simulink model "HVDCMMCInterconnection"  (R2023b)
settings: Solver=FixedStepDiscrete  StartTime=0.0  StopTime=10  FixedStep=Ts_Power  RelTol=1e-4
PreLoadFcn:
  | HVDCMMCInterconnectionParam
StartFcn:
  | tic
StopFcn:
  | toc
values from neighbouring files (symbols this model uses):
  C_PM = 1.758e-3    (= 0.001758)    [HVDCMMCInterconnectionParam.m]
  Cg = 50e-9    (= 5e-08)    [HVDCMMCInterconnectionParam.m]
  D_R = 0.001    [HVDCMMCInterconnectionParam.m]
  D_Rs = 1e8    (= 100000000)    [HVDCMMCInterconnectionParam.m]
  D_Vf = 0    [HVDCMMCInterconnectionParam.m]
  Fnom = 50    [HVDCMMCInterconnectionParam.m]
  HRM = 2    [HVDCMMCInterconnectionParam.m]
  Ki_Ireg = 6    [HVDCMMCInterconnectionParam.m]
  Ki_Preg = 1.0    (= 1)    [HVDCMMCInterconnectionParam.m]
  Ki_Qreg = 1.0    (= 1)    [HVDCMMCInterconnectionParam.m]
  Ki_VDCreg = 100    [HVDCMMCInterconnectionParam.m]
  Kp_Ireg = 0.6    [HVDCMMCInterconnectionParam.m]
  Kp_Preg = 0.5/3    (= 0.166666666667)    [HVDCMMCInterconnectionParam.m]
  Kp_Qreg = 0.5/3    (= 0.166666666667)    [HVDCMMCInterconnectionParam.m]
  Kp_VDCreg = 4    [HVDCMMCInterconnectionParam.m]
  L_cable = 15e-3    (= 0.015)    [HVDCMMCInterconnectionParam.m]
  Larm = Larm_pu*(Zb_ac/(2*pi*Fnom))    [HVDCMMCInterconnectionParam.m]
  Lff = Larm_pu/2    (= 0.075)    [HVDCMMCInterconnectionParam.m]
  Limits_Ireg = [ 2.0  -2.0]    [HVDCMMCInterconnectionParam.m]
  Limits_Preg = [ 1.2, 0.8 ]    [HVDCMMCInterconnectionParam.m]
  Limits_Qreg = [ 0.25, -0.25 ]    [HVDCMMCInterconnectionParam.m]
  Limits_VDCreg = [ 2.0  -2.0]    [HVDCMMCInterconnectionParam.m]
  Lxfo = 0.12    [HVDCMMCInterconnectionParam.m]
  Nb_PM = 36    [HVDCMMCInterconnectionParam.m]
  Pnom = 1000e6    (= 1000000000)    [HVDCMMCInterconnectionParam.m]
  R_cable = 0.5    [HVDCMMCInterconnectionParam.m]
  R_startup = 400    [HVDCMMCInterconnectionParam.m]
  Rarm = Rarm_pu*Zb_ac    [HVDCMMCInterconnectionParam.m]
  Rff = Rarm_pu/2    (= 0.00075)    [HVDCMMCInterconnectionParam.m]
  Rg = 100    [HVDCMMCInterconnectionParam.m]
  Rxfo = 0.003    [HVDCMMCInterconnectionParam.m]
  Slope_Pref = 0.5    [HVDCMMCInterconnectionParam.m]
  Slope_Qref = 0.5    [HVDCMMCInterconnectionParam.m]
  Slope_Vdc_ref = Vnom_dc/5    (= 128000)    [HVDCMMCInterconnectionParam.m]
  Tbrk1_On = 0.1    [HVDCMMCInterconnectionParam.m]
  Tbrk2_On = 1.0    (= 1)    [HVDCMMCInterconnectionParam.m]
  Tdeblock = 1.5    [HVDCMMCInterconnectionParam.m]
  Tfault = 9999    [HVDCMMCInterconnectionParam.m]
  Ton_Converter2 = 4    [HVDCMMCInterconnectionParam.m]
  Ton_PQreg = 4    [HVDCMMCInterconnectionParam.m]
  Ton_VDCreg = 1.5    [HVDCMMCInterconnectionParam.m]
  Ts = Ts_Control    (= 4e-05)    [HVDCMMCInterconnectionParam.m]    (also in power_circ2ss_sps_calc.m = 1e-06)
  Ts_Control = 40e-6    (= 4e-05)    [HVDCMMCInterconnectionParam.m]
  Ts_Power = 20e-6    (= 2e-05)    [HVDCMMCInterconnectionParam.m]
  Vb_ac = sqrt(2/3)*Vnom_sec    [HVDCMMCInterconnectionParam.m]
  Vb_dc = Vnom_dc    (= 640000)    [HVDCMMCInterconnectionParam.m]
  Vc0_PM = 0    [HVDCMMCInterconnectionParam.m]
  Vnom_dc = 640e3    (= 640000)    [HVDCMMCInterconnectionParam.m]
  Vnom_prim = 400e3    (= 400000)    [HVDCMMCInterconnectionParam.m]
  Vnom_sec = 333e3    (= 333000)    [HVDCMMCInterconnectionParam.m]
  w = 2*pi*Fnom    (= 314.159265359)    [HVDCMMCInterconnectionParam.m]
undefined symbols (not defined in the file or in its folder): ACDC, ACDC3, DiscIntNeverNeededParam, gcbh, Pcc, S, sps_AC, sps_rtmsupport
libraries: simulink x61, spsControlledVoltageSourceLib x56, spsCurrentMeasurementLib x56, spsDiodeLib x40, spsSeriesRLCBranchLib x32, spsVoltageMeasurementLib x20, powerlib_extras x9, spsHalfBridgeMMCmodel x8, spsGroundLib x7, spsSecondOrderFilterLib x6, spsabctodq0Lib x6, spsMeanLib x3
(part 11 of 11)

== system HVDCMMCInterconnection/DSS1/U-I3/MUX1 ==
  In1 : Inport
  In2 : Inport  Port=2
  Demux4 : Demux  Outputs=3
  Demux5 : Demux  Outputs=3
  Mux13 : Mux  Inputs=2
  Mux14 : Mux  Inputs=2
  Mux15 : Mux  Inputs=3
  Mux8 : Mux  Inputs=2
  Sum1 : Sum  Inputs=1  InputSameDT=on  SaturateOnIntegerOverflow=on  OutDataTypeStr=Inherit: Same as first input
  Sum4 : Sum  Inputs=1  InputSameDT=on  SaturateOnIntegerOverflow=on  OutDataTypeStr=Inherit: Same as first input
  Sum5 : Sum  Inputs=1  InputSameDT=on  SaturateOnIntegerOverflow=on  OutDataTypeStr=Inherit: Same as first input
  UBrk1_EMT : Outport
  wires:
  Demux5/3 -> Mux14/2
  In1/1 -> Demux4/1
  Demux4/1 -> Mux8/1
  Demux5/1 -> Mux8/2
  In2/1 -> Demux5/1
  Sum1/1 -> Mux15/1
  Demux5/2 -> Mux13/2
  Mux14/1 -> Sum5/1
  Mux8/1 -> Sum1/1
  Demux4/2 -> Mux13/1
  Mux13/1 -> Sum4/1
  Sum5/1 -> Mux15/3
  Sum4/1 -> Mux15/2
  Demux4/3 -> Mux14/1
  Mux15/1 -> UBrk1_EMT/1

== system HVDCMMCInterconnection/DSS1/U-I3/MUX2 ==
  In1 : Inport
  In2 : Inport  Port=2
  Demux4 : Demux  Outputs=3
  Demux5 : Demux  Outputs=3
  Mux13 : Mux  Inputs=2
  Mux14 : Mux  Inputs=2
  Mux15 : Mux  Inputs=3
  Mux8 : Mux  Inputs=2
  Sum1 : Sum  Inputs=1  InputSameDT=on  SaturateOnIntegerOverflow=on  OutDataTypeStr=Inherit: Same as first input
  Sum4 : Sum  Inputs=1  InputSameDT=on  SaturateOnIntegerOverflow=on  OutDataTypeStr=Inherit: Same as first input
  Sum5 : Sum  Inputs=1  InputSameDT=on  SaturateOnIntegerOverflow=on  OutDataTypeStr=Inherit: Same as first input
  UBrk1_EMT : Outport
  wires:
  Demux5/3 -> Mux14/2
  In1/1 -> Demux4/1
  Demux4/1 -> Mux8/1
  Demux5/1 -> Mux8/2
  In2/1 -> Demux5/1
  Sum1/1 -> Mux15/1
  Demux5/2 -> Mux13/2
  Mux14/1 -> Sum5/1
  Mux8/1 -> Sum1/1
  Demux4/2 -> Mux13/1
  Mux13/1 -> Sum4/1
  Sum5/1 -> Mux15/3
  Sum4/1 -> Mux15/2
  Demux4/3 -> Mux14/1
  Mux15/1 -> UBrk1_EMT/1

== system HVDCMMCInterconnection/DSS2/BRK_CTRL1/MUX2 ==
  In1 : Inport
  In2 : Inport  Port=2
  Demux4 : Demux  Outputs=3
  Demux5 : Demux  Outputs=3
  Mux13 : Mux  Inputs=2
  Mux14 : Mux  Inputs=2
  Mux15 : Mux  Inputs=3
  Mux8 : Mux  Inputs=2
  Sum1 : Sum  Inputs=1  InputSameDT=on  SaturateOnIntegerOverflow=on  OutDataTypeStr=Inherit: Same as first input
  Sum4 : Sum  Inputs=1  InputSameDT=on  SaturateOnIntegerOverflow=on  OutDataTypeStr=Inherit: Same as first input
  Sum5 : Sum  Inputs=1  InputSameDT=on  SaturateOnIntegerOverflow=on  OutDataTypeStr=Inherit: Same as first input
  Out1 : Outport
  wires:
  Demux5/3 -> Mux14/2
  In1/1 -> Demux4/1
  Demux4/1 -> Mux8/1
  Demux5/1 -> Mux8/2
  In2/1 -> Demux5/1
  Sum1/1 -> Mux15/1
  Demux5/2 -> Mux13/2
  Mux14/1 -> Sum5/1
  Mux8/1 -> Sum1/1
  Demux4/2 -> Mux13/1
  Mux13/1 -> Sum4/1
  Sum5/1 -> Mux15/3
  Sum4/1 -> Mux15/2
  Demux4/3 -> Mux14/1
  Mux15/1 -> Out1/1

== system HVDCMMCInterconnection/DSS2/BRK_CTRL3/MUX2 ==
  In1 : Inport
  In2 : Inport  Port=2
  Demux4 : Demux  Outputs=3
  Demux5 : Demux  Outputs=3
  Mux13 : Mux  Inputs=2
  Mux14 : Mux  Inputs=2
  Mux15 : Mux  Inputs=3
  Mux8 : Mux  Inputs=2
  Sum1 : Sum  Inputs=1  InputSameDT=on  SaturateOnIntegerOverflow=on  OutDataTypeStr=Inherit: Same as first input
  Sum4 : Sum  Inputs=1  InputSameDT=on  SaturateOnIntegerOverflow=on  OutDataTypeStr=Inherit: Same as first input
  Sum5 : Sum  Inputs=1  InputSameDT=on  SaturateOnIntegerOverflow=on  OutDataTypeStr=Inherit: Same as first input
  Out1 : Outport
  wires:
  Demux5/3 -> Mux14/2
  In1/1 -> Demux4/1
  Demux4/1 -> Mux8/1
  Demux5/1 -> Mux8/2
  In2/1 -> Demux5/1
  Sum1/1 -> Mux15/1
  Demux5/2 -> Mux13/2
  Mux14/1 -> Sum5/1
  Mux8/1 -> Sum1/1
  Demux4/2 -> Mux13/1
  Mux13/1 -> Sum4/1
  Sum5/1 -> Mux15/3
  Sum4/1 -> Mux15/2
  Demux4/3 -> Mux14/1
  Mux15/1 -> Out1/1

== system HVDCMMCInterconnection/DSS2/U-I1/MUX1 ==
  In1 : Inport
  In2 : Inport  Port=2
  Demux4 : Demux  Outputs=3
  Demux5 : Demux  Outputs=3
  Mux13 : Mux  Inputs=2
  Mux14 : Mux  Inputs=2
  Mux15 : Mux  Inputs=3
  Mux8 : Mux  Inputs=2
  Sum1 : Sum  Inputs=1  InputSameDT=on  SaturateOnIntegerOverflow=on  OutDataTypeStr=Inherit: Same as first input
  Sum4 : Sum  Inputs=1  InputSameDT=on  SaturateOnIntegerOverflow=on  OutDataTypeStr=Inherit: Same as first input
  Sum5 : Sum  Inputs=1  InputSameDT=on  SaturateOnIntegerOverflow=on  OutDataTypeStr=Inherit: Same as first input
  UBrk1_EMT : Outport
  wires:
  Demux5/3 -> Mux14/2
  In1/1 -> Demux4/1
  Demux4/1 -> Mux8/1
  Demux5/1 -> Mux8/2
  In2/1 -> Demux5/1
  Sum1/1 -> Mux15/1
  Demux5/2 -> Mux13/2
  Mux14/1 -> Sum5/1
  Mux8/1 -> Sum1/1
  Demux4/2 -> Mux13/1
  Mux13/1 -> Sum4/1
  Sum5/1 -> Mux15/3
  Sum4/1 -> Mux15/2
  Demux4/3 -> Mux14/1
  Mux15/1 -> UBrk1_EMT/1

== system HVDCMMCInterconnection/DSS2/U-I1/MUX2 ==
  In1 : Inport
  In2 : Inport  Port=2
  Demux4 : Demux  Outputs=3
  Demux5 : Demux  Outputs=3
  Mux13 : Mux  Inputs=2
  Mux14 : Mux  Inputs=2
  Mux15 : Mux  Inputs=3
  Mux8 : Mux  Inputs=2
  Sum1 : Sum  Inputs=1  InputSameDT=on  SaturateOnIntegerOverflow=on  OutDataTypeStr=Inherit: Same as first input
  Sum4 : Sum  Inputs=1  InputSameDT=on  SaturateOnIntegerOverflow=on  OutDataTypeStr=Inherit: Same as first input
  Sum5 : Sum  Inputs=1  InputSameDT=on  SaturateOnIntegerOverflow=on  OutDataTypeStr=Inherit: Same as first input
  UBrk1_EMT : Outport
  wires:
  Demux5/3 -> Mux14/2
  In1/1 -> Demux4/1
  Demux4/1 -> Mux8/1
  Demux5/1 -> Mux8/2
  In2/1 -> Demux5/1
  Sum1/1 -> Mux15/1
  Demux5/2 -> Mux13/2
  Mux14/1 -> Sum5/1
  Mux8/1 -> Sum1/1
  Demux4/2 -> Mux13/1
  Mux13/1 -> Sum4/1
  Sum5/1 -> Mux15/3
  Sum4/1 -> Mux15/2
  Demux4/3 -> Mux14/1
  Mux15/1 -> UBrk1_EMT/1

== system HVDCMMCInterconnection/DSS2/U-I2/BRK_CTRL3 ==
  UBrk1_EMT : Inport
  Brk_ON : Inport  Port=2
  Cast To Double{,1..3} (4 alike) : DataTypeConversion  OutDataTypeStr=double  SaturateOnIntegerOverflow=off  RndMeth=Floor
  Compare To Constant4 : simulink/Logic and Bit Operations/Compare To Constant  relop=>  const=0  OutDataTypeStr=boolean
  Gain : Gain  Gain=1/1e6
  Gain3 : Gain  Gain=1/0.01
  MUX2 : Subsystem
  NOT2 : Logic  Operator=NOT  IconShape=distinctive  AllPortsSameDT=off  OutDataTypeStr=boolean
  Product : Product
  Product1 : Product
  IBrk1_ss : Outport
  wires:
  Cast To Double1/1 -> Product/2
  Product1/1 -> MUX2/2(In2)
  UBrk1_EMT/1 -> Gain3/1, Gain/1
  Compare To Constant4/1 -> Cast To Double1/1, NOT2/1
  Product/1 -> MUX2/1(In1)
  Gain/1 -> Cast To Double3/1
  NOT2/1 -> Cast To Double2/1
  Cast To Double/1 -> Product/1
  Gain3/1 -> Cast To Double/1
  Cast To Double3/1 -> Product1/2
  Brk_ON/1 -> Compare To Constant4/1
  Cast To Double2/1 -> Product1/1
  MUX2/1(Out1) -> IBrk1_ss/1  "IBrk1_ss"

== system HVDCMMCInterconnection/DSS2/U-I2/MUX1 ==
  In1 : Inport
  In2 : Inport  Port=2
  Demux4 : Demux  Outputs=3
  Demux5 : Demux  Outputs=3
  Mux13 : Mux  Inputs=2
  Mux14 : Mux  Inputs=2
  Mux15 : Mux  Inputs=3
  Mux8 : Mux  Inputs=2
  Sum1 : Sum  Inputs=1  InputSameDT=on  SaturateOnIntegerOverflow=on  OutDataTypeStr=Inherit: Same as first input
  Sum4 : Sum  Inputs=1  InputSameDT=on  SaturateOnIntegerOverflow=on  OutDataTypeStr=Inherit: Same as first input
  Sum5 : Sum  Inputs=1  InputSameDT=on  SaturateOnIntegerOverflow=on  OutDataTypeStr=Inherit: Same as first input
  UBrk1_EMT : Outport
  wires:
  Demux5/3 -> Mux14/2
  In1/1 -> Demux4/1
  Demux4/1 -> Mux8/1
  Demux5/1 -> Mux8/2
  In2/1 -> Demux5/1
  Sum1/1 -> Mux15/1
  Demux5/2 -> Mux13/2
  Mux14/1 -> Sum5/1
  Mux8/1 -> Sum1/1
  Demux4/2 -> Mux13/1
  Mux13/1 -> Sum4/1
  Sum5/1 -> Mux15/3
  Sum4/1 -> Mux15/2
  Demux4/3 -> Mux14/1
  Mux15/1 -> UBrk1_EMT/1

== system HVDCMMCInterconnection/DSS2/U-I2/MUX2 ==
  In1 : Inport
  In2 : Inport  Port=2
  Demux4 : Demux  Outputs=3
  Demux5 : Demux  Outputs=3
  Mux13 : Mux  Inputs=2
  Mux14 : Mux  Inputs=2
  Mux15 : Mux  Inputs=3
  Mux8 : Mux  Inputs=2
  Sum1 : Sum  Inputs=1  InputSameDT=on  SaturateOnIntegerOverflow=on  OutDataTypeStr=Inherit: Same as first input
  Sum4 : Sum  Inputs=1  InputSameDT=on  SaturateOnIntegerOverflow=on  OutDataTypeStr=Inherit: Same as first input
  Sum5 : Sum  Inputs=1  InputSameDT=on  SaturateOnIntegerOverflow=on  OutDataTypeStr=Inherit: Same as first input
  UBrk1_EMT : Outport
  wires:
  Demux5/3 -> Mux14/2
  In1/1 -> Demux4/1
  Demux4/1 -> Mux8/1
  Demux5/1 -> Mux8/2
  In2/1 -> Demux5/1
  Sum1/1 -> Mux15/1
  Demux5/2 -> Mux13/2
  Mux14/1 -> Sum5/1
  Mux8/1 -> Sum1/1
  Demux4/2 -> Mux13/1
  Mux13/1 -> Sum4/1
  Sum5/1 -> Mux15/3
  Sum4/1 -> Mux15/2
  Demux4/3 -> Mux14/1
  Mux15/1 -> UBrk1_EMT/1

== system HVDCMMCInterconnection/MMC/Ap/Diode2 ==
  Diode : PMComponent  PhysicalDomain=powersysdomain  LeftPortType=p1  RightPortType=p1  LConnTagsString=a  RConnTagsString=__new0  mask(InnerPowersysBlock){}
      mask Display: disp('SPS internal use\nDo not delete')
  ISWITCH : Terminator
  Model : spsDiodeModel/Discrete  SystemSampleTime=-1  VariantActivationTime=update diagram  AllowFlexibleInterface=on  Latency=0  AutoFrameSizeCalculation=off
  VF : Terminator
  a : PMIOPort  Side=Left
  k : PMIOPort  Port=2  Side=Right
  m : Outport  VectorParamsAs1DForOutWhenUnconnected=off
  tag scope: T41_3630_2436379962024=global
  wires:
  Model/2 -> m/1
  [T43_3865_3018745695692] -> Model/2
  Model/3 -> VF/1
  Model/4 -> [T41_3630_2436379962024]
  Model/1 -> ISWITCH/1
  [T44_3964_3123742533462] -> Model/1
  connections:
  Diode/RConn1 -- k/RConn1
  a/RConn1 -- Diode/LConn1

== system HVDCMMCInterconnection/MMC1/Ap/Diode2 ==
  Diode : PMComponent  PhysicalDomain=powersysdomain  LeftPortType=p1  RightPortType=p1  LConnTagsString=a  RConnTagsString=__new0  mask(InnerPowersysBlock){}
      mask Display: disp('SPS internal use\nDo not delete')
  ISWITCH : Terminator
  Model : spsDiodeModel/Discrete  SystemSampleTime=-1  VariantActivationTime=update diagram  AllowFlexibleInterface=on  Latency=0  AutoFrameSizeCalculation=off
  VF : Terminator
  a : PMIOPort  Side=Left
  k : PMIOPort  Port=2  Side=Right
  m : Outport  VectorParamsAs1DForOutWhenUnconnected=off
  tag scope: T42_3679_2536778320488=global
  wires:
  Model/2 -> m/1
  [T44_3914_3147049646697] -> Model/2
  Model/3 -> VF/1
  Model/4 -> [T42_3679_2536778320488]
  Model/1 -> ISWITCH/1
  [T45_4013_3259919479727] -> Model/1
  connections:
  Diode/RConn1 -- k/RConn1
  a/RConn1 -- Diode/LConn1

== system HVDCMMCInterconnection/DSS/U-I2/BRK_CTRL3/MUX2 ==
  In1 : Inport
  In2 : Inport  Port=2
  Demux4 : Demux  Outputs=3
  Demux5 : Demux  Outputs=3
  Mux13 : Mux  Inputs=2
  Mux14 : Mux  Inputs=2
  Mux15 : Mux  Inputs=3
  Mux8 : Mux  Inputs=2
  Sum1 : Sum  Inputs=1  InputSameDT=on  SaturateOnIntegerOverflow=on  OutDataTypeStr=Inherit: Same as first input
  Sum4 : Sum  Inputs=1  InputSameDT=on  SaturateOnIntegerOverflow=on  OutDataTypeStr=Inherit: Same as first input
  Sum5 : Sum  Inputs=1  InputSameDT=on  SaturateOnIntegerOverflow=on  OutDataTypeStr=Inherit: Same as first input
  Out1 : Outport
  wires:
  Demux5/3 -> Mux14/2
  In1/1 -> Demux4/1
  Demux4/1 -> Mux8/1
  Demux5/1 -> Mux8/2
  In2/1 -> Demux5/1
  Sum1/1 -> Mux15/1
  Demux5/2 -> Mux13/2
  Mux14/1 -> Sum5/1
  Mux8/1 -> Sum1/1
  Demux4/2 -> Mux13/1
  Mux13/1 -> Sum4/1
  Sum5/1 -> Mux15/3
  Sum4/1 -> Mux15/2
  Demux4/3 -> Mux14/1
  Mux15/1 -> Out1/1

== system HVDCMMCInterconnection/DSS1/U-I2/BRK_CTRL3/MUX2 ==
  In1 : Inport
  In2 : Inport  Port=2
  Demux4 : Demux  Outputs=3
  Demux5 : Demux  Outputs=3
  Mux13 : Mux  Inputs=2
  Mux14 : Mux  Inputs=2
  Mux15 : Mux  Inputs=3
  Mux8 : Mux  Inputs=2
  Sum1 : Sum  Inputs=1  InputSameDT=on  SaturateOnIntegerOverflow=on  OutDataTypeStr=Inherit: Same as first input
  Sum4 : Sum  Inputs=1  InputSameDT=on  SaturateOnIntegerOverflow=on  OutDataTypeStr=Inherit: Same as first input
  Sum5 : Sum  Inputs=1  InputSameDT=on  SaturateOnIntegerOverflow=on  OutDataTypeStr=Inherit: Same as first input
  Out1 : Outport
  wires:
  Demux5/3 -> Mux14/2
  In1/1 -> Demux4/1
  Demux4/1 -> Mux8/1
  Demux5/1 -> Mux8/2
  In2/1 -> Demux5/1
  Sum1/1 -> Mux15/1
  Demux5/2 -> Mux13/2
  Mux14/1 -> Sum5/1
  Mux8/1 -> Sum1/1
  Demux4/2 -> Mux13/1
  Mux13/1 -> Sum4/1
  Sum5/1 -> Mux15/3
  Sum4/1 -> Mux15/2
  Demux4/3 -> Mux14/1
  Mux15/1 -> Out1/1

== system HVDCMMCInterconnection/DSS2/U-I2/BRK_CTRL3/MUX2 ==
  In1 : Inport
  In2 : Inport  Port=2
  Demux4 : Demux  Outputs=3
  Demux5 : Demux  Outputs=3
  Mux13 : Mux  Inputs=2
  Mux14 : Mux  Inputs=2
  Mux15 : Mux  Inputs=3
  Mux8 : Mux  Inputs=2
  Sum1 : Sum  Inputs=1  InputSameDT=on  SaturateOnIntegerOverflow=on  OutDataTypeStr=Inherit: Same as first input
  Sum4 : Sum  Inputs=1  InputSameDT=on  SaturateOnIntegerOverflow=on  OutDataTypeStr=Inherit: Same as first input
  Sum5 : Sum  Inputs=1  InputSameDT=on  SaturateOnIntegerOverflow=on  OutDataTypeStr=Inherit: Same as first input
  Out1 : Outport
  wires:
  Demux5/3 -> Mux14/2
  In1/1 -> Demux4/1
  Demux4/1 -> Mux8/1
  Demux5/1 -> Mux8/2
  In2/1 -> Demux5/1
  Sum1/1 -> Mux15/1
  Demux5/2 -> Mux13/2
  Mux14/1 -> Sum5/1
  Mux8/1 -> Sum1/1
  Demux4/2 -> Mux13/1
  Mux13/1 -> Sum4/1
  Sum5/1 -> Mux15/3
  Sum4/1 -> Mux15/2
  Demux4/3 -> Mux14/1
  Mux15/1 -> Out1/1

== matlab function HVDCMMCInterconnection/MATLAB Function4 ==
  data: u input; y output [1..100]; Ad parameter; Bd parameter; Cd parameter; Dd parameter; swOnRes parameter; swOffRes parameter; swType parameter; brkVec input
function y  = fDSS(u, Ad, Bd, Cd, Dd, swOnRes, swOffRes, swType, brkVec)

% INIT
x = zeros(size(Ad,1),1);
y = zeros(size(Cd,1),1);

persistent Ad11;
persistent Ad12;
persistent Ad21;
persistent Ad22;

persistent Bd11;
persistent Bd12;
persistent Bd21;
persistent Bd22;
persistent Cd11;
persistent Cd12;
persistent Cd21;
persistent Cd22;
persistent Dd11;
persistent Dd12;
persistent Dd21;
persistent Dd22;

persistent Ads;
persistent Bds;
persistent Cds;
persistent Dds;

persistent x_old;
persistent swVec;
persistent swVecOld;

persistent nrSt;
persistent nrOut;

persistent nsw;
persistent ncb;
persistent npe;

persistent kb;


if(isempty(x_old))
    nrSt = size(Ad,1);
    nrOut = size(Cd,1);

    ncb = sum(swType==1) + sum(swType==2);
    npe = sum(swType==3);
    nsw = ncb + npe;
    
    Ad11 = Ad(1:nsw,1:nsw);         if(isempty(Ad11)) Ad11 = zeros(3,3); end
    Ad12 = Ad(1:nsw,nsw+1:end);     if(isempty(Ad12)) Ad12 = zeros(3,3); end
    Ad21 = Ad(nsw+1:end,1:nsw);     if(isempty(Ad21)) Ad21 = zeros(3,3); end
    Ad22 = Ad(nsw+1:end,nsw+1:end); if(isempty(Ad22)) Ad22 = zeros(3,3); end

    Bd11 = Bd(1:nsw,1:nsw);         if(isempty(Bd11)) Bd11 = zeros(3,3); end
    Bd12 = Bd(1:nsw,nsw+1:end);     if(isempty(Bd12)) Bd12 = zeros(3,3); end
    Bd21 = Bd(nsw+1:end,1:nsw);     if(isempty(Bd21)) Bd21 = zeros(3,3); end
    Bd22 = Bd(nsw+1:end,nsw+1:end); if(isempty(Bd22)) Bd22 = zeros(3,size(Bd,2)-nsw); end

    Cd11 = Cd(1:nsw,1:nsw);         if(isempty(Cd11)) Cd11 = zeros(3,3); end
    Cd12 = Cd(1:nsw,nsw+1:end);     if(isempty(Cd12)) Cd12 = zeros(3,3); end
    Cd21 = Cd(nsw+1:end,1:nsw);     if(isempty(Cd21)) Cd21 = zeros(3,3); end
    Cd22 = Cd(nsw+1:end,nsw+1:end); if(isempty(Cd22)) Cd22 = zeros(size(Cd,1)-nsw,size(Cd,2)); end

    Dd11 = Dd(1:nsw,1:nsw);         if(isempty(Dd11)) Dd11 = zeros(3,3); end
    Dd12 = Dd(1:nsw,nsw+1:end);     if(isempty(Dd12)) Dd12 = zeros(3,3); end
    Dd21 = Dd(nsw+1:end,1:nsw);     if(isempty(Dd21)) Dd21 = zeros(3,3); end
    Dd22 = Dd(nsw+1:end,nsw+1:end); if(isempty(Dd22)) Dd22 = zeros(3,3); end

    x_old = zeros(size(Ad,1),1);

    swVec = [brkVec; zeros(nsw - ncb,1) ]; 
    swVecOld = zeros(nsw,1); 

    kb = swOffRes.*abs(1-swVec)+swOnRes.*abs(0-swVec);

    Dd11k = zeros(size(Dd11)); for i = 1 : nsw, Dd11k(:,i) = Dd11(:,i)/kb(i); end
    D11Ik = eye(nsw)/(eye(nsw) - Dd11k);

    Dd21k = zeros(size(Dd21)); for i = 1 : nsw, Dd21k(:,i) = Dd21(:,i)/kb(i);  end

    E = D11Ik * Cd11;
    F = D11Ik * Cd12;
    I = D11Ik*Dd12;

    Bd11k = zeros(size(Bd11)); for i = 1 : nsw, Bd11k(:,i) = Bd11(:,i)/kb(i);  end
    Bd21k = zeros(size(Bd21)); for i = 1 : nsw, Bd21k(:,i) = Bd21(:,i)/kb(i);  end

    Ads = [Ad11+Bd11k*E Ad12+Bd11k*F ; Ad21+Bd21k*E Ad22+Bd21k*F ];
    Bds = [(Bd11k*I + Bd12); Bd21k*I + Bd22];
    Cds = [ D11Ik * Cd11 D11Ik * Cd12 ; Dd21k*D11Ik*Cd11 + Cd21 Dd21k*D11Ik*Cd12 + Cd22];
    Dds = [ D11Ik*Dd12; (Dd22+Dd21k*D11Ik*Dd12)];

end

%is = zeros(nsw,1);

swVec(1:ncb) = brkVec(1:ncb);

if(any(swVecOld ~= swVec))

    kb = swOffRes.*abs(1-swVec)+swOnRes.*abs(0-swVec);
    Dd11k = zeros(size(Dd11)); for i = 1 : nsw, Dd11k(:,i) = Dd11(:,i)/kb(i); end
    D11Ik = eye(nsw)/(eye(nsw) - Dd11k);

    Dd21k = zeros(size(Dd21)); for i = 1 : nsw, Dd21k(:,i) = Dd21(:,i)/kb(i);  end

    E = D11Ik * Cd11;
    F = D11Ik * Cd12;
    I = D11Ik * Dd12;

    Bd11k = zeros(size(Bd11)); for i = 1 : nsw, Bd11k(:,i) = Bd11(:,i)/kb(i);  end
    Bd21k = zeros(size(Bd21)); for i = 1 : nsw, Bd21k(:,i) = Bd21(:,i)/kb(i);  end

    Ads = [Ad11+Bd11k*E Ad12+Bd11k*F ; Ad21+Bd21k*E Ad22+Bd21k*F ];
    Bds = [(Bd11k*I + Bd12); Bd21k*I + Bd22];
    Cds = [ D11Ik * Cd11 D11Ik * Cd12 ; Dd21k*D11Ik*Cd11 + Cd21 Dd21k*D11Ik*Cd12 + Cd22];
    Dds = [ D11Ik*Dd12; (Dd22+Dd21k*D11Ik*Dd12)];
end

swVecOld = swVec;


    x           = Ads*x_old  + Bds*u(nsw+1:end);  x_old(1:nrSt) = x(1:nrSt);                                                   
    y(1:nrOut)  = Cds*x      + Dds*u(nsw+1:end);        


    is = y(1:nsw)./kb'; %Calculate switch currents


    for i = ncb:nsw

        if(i > ncb) %Breakers

            if(swVec(i)==1 && (is(i) <= eps))
                swVec(i) = 0; %Open
            end

            if(swVec(i)==0 && y(i) > 0)
                swVec(i) = 1; %Close
            end
        end

    end




end

== matlab function HVDCMMCInterconnection/MATLAB Function5 ==
  data: u input; y output [1..100]; Ad parameter; Bd parameter; Cd parameter; Dd parameter; swOnRes parameter; swOffRes parameter; swType parameter; brkVec input; status output
function [y, status]  = fDSS(u, Ad, Bd, Cd, Dd, swOnRes, swOffRes, swType, brkVec)

% INIT
x = zeros(size(Ad,1),1);
y = zeros(size(Cd,1),1);


persistent Ad11;
persistent Ad12;
persistent Ad21;
persistent Ad22;

persistent Bd11;
persistent Bd12;
persistent Bd21;
persistent Bd22;
persistent Cd11;
persistent Cd12;
persistent Cd21;
persistent Cd22;
persistent Dd11;
persistent Dd12;
persistent Dd21;
persistent Dd22;

persistent Ads;
persistent Bds;
persistent Cds;
persistent Dds;

persistent x_old;
persistent swVec;
persistent swVecOld;

persistent nrSt;
persistent nrOut;

persistent nsw;
persistent ncb;
persistent npe;

persistent kb;


if(isempty(x_old))
    nrSt = size(Ad,1);
    nrOut = size(Cd,1);

    ncb = sum(swType==1) + sum(swType==2);
    npe = sum(swType==3);
    nsw = ncb + npe;
    
    Ad11 = Ad(1:nsw,1:nsw);         if(isempty(Ad11)) Ad11 = zeros(3,3); end
    Ad12 = Ad(1:nsw,nsw+1:end);     if(isempty(Ad12)) Ad12 = zeros(3,3); end
    Ad21 = Ad(nsw+1:end,1:nsw);     if(isempty(Ad21)) Ad21 = zeros(3,3); end
    Ad22 = Ad(nsw+1:end,nsw+1:end); if(isempty(Ad22)) Ad22 = zeros(3,3); end

    Bd11 = Bd(1:nsw,1:nsw);         if(isempty(Bd11)) Bd11 = zeros(3,3); end
    Bd12 = Bd(1:nsw,nsw+1:end);     if(isempty(Bd12)) Bd12 = zeros(3,3); end
    Bd21 = Bd(nsw+1:end,1:nsw);     if(isempty(Bd21)) Bd21 = zeros(3,3); end
    Bd22 = Bd(nsw+1:end,nsw+1:end); if(isempty(Bd22)) Bd22 = zeros(3,size(Bd,2)-nsw); end

    Cd11 = Cd(1:nsw,1:nsw);         if(isempty(Cd11)) Cd11 = zeros(3,3); end
    Cd12 = Cd(1:nsw,nsw+1:end);     if(isempty(Cd12)) Cd12 = zeros(3,3); end
    Cd21 = Cd(nsw+1:end,1:nsw);     if(isempty(Cd21)) Cd21 = zeros(3,3); end
    Cd22 = Cd(nsw+1:end,nsw+1:end); if(isempty(Cd22)) Cd22 = zeros(size(Cd,1)-nsw,size(Cd,2)); end

    Dd11 = Dd(1:nsw,1:nsw);         if(isempty(Dd11)) Dd11 = zeros(3,3); end
    Dd12 = Dd(1:nsw,nsw+1:end);     if(isempty(Dd12)) Dd12 = zeros(3,3); end
    Dd21 = Dd(nsw+1:end,1:nsw);     if(isempty(Dd21)) Dd21 = zeros(3,3); end
    Dd22 = Dd(nsw+1:end,nsw+1:end); if(isempty(Dd22)) Dd22 = zeros(3,3); end

    x_old = zeros(size(Ad,1),1);

    swVec = [brkVec; zeros(nsw - ncb,1) ]; 
    swVecOld = zeros(nsw,1); 

    kb = swOffRes.*abs(1-swVec)+swOnRes.*abs(0-swVec);

    Dd11k = zeros(size(Dd11)); for i = 1 : nsw, Dd11k(:,i) = Dd11(:,i)/kb(i); end
    D11Ik = eye(nsw)/(eye(nsw) - Dd11k);

    Dd21k = zeros(size(Dd21)); for i = 1 : nsw, Dd21k(:,i) = Dd21(:,i)/kb(i);  end

    E = D11Ik * Cd11;
    F = D11Ik * Cd12;
    I = D11Ik*Dd12;

    Bd11k = zeros(size(Bd11)); for i = 1 : nsw, Bd11k(:,i) = Bd11(:,i)/kb(i);  end
    Bd21k = zeros(size(Bd21)); for i = 1 : nsw, Bd21k(:,i) = Bd21(:,i)/kb(i);  end

    Ads = [Ad11+Bd11k*E Ad12+Bd11k*F ; Ad21+Bd21k*E Ad22+Bd21k*F ];
    Bds = [(Bd11k*I + Bd12); Bd21k*I + Bd22];
    Cds = [ D11Ik * Cd11 D11Ik * Cd12 ; Dd21k*D11Ik*Cd11 + Cd21 Dd21k*D11Ik*Cd12 + Cd22];
    Dds = [ D11Ik*Dd12; (Dd22+Dd21k*D11Ik*Dd12)];

end

status = zeros(size(swType));

%is = zeros(nsw,1);

swVec(1:ncb) = brkVec(1:ncb);

if(any(swVecOld ~= swVec))

    kb = swOffRes.*abs(1-swVec)+swOnRes.*abs(0-swVec);
    Dd11k = zeros(size(Dd11)); for i = 1 : nsw, Dd11k(:,i) = Dd11(:,i)/kb(i); end
    D11Ik = eye(nsw)/(eye(nsw) - Dd11k);

    Dd21k = zeros(size(Dd21)); for i = 1 : nsw, Dd21k(:,i) = Dd21(:,i)/kb(i);  end

    E = D11Ik * Cd11;
    F = D11Ik * Cd12;
    I = D11Ik * Dd12;

    Bd11k = zeros(size(Bd11)); for i = 1 : nsw, Bd11k(:,i) = Bd11(:,i)/kb(i);  end
    Bd21k = zeros(size(Bd21)); for i = 1 : nsw, Bd21k(:,i) = Bd21(:,i)/kb(i);  end

    Ads = [Ad11+Bd11k*E Ad12+Bd11k*F ; Ad21+Bd21k*E Ad22+Bd21k*F ];
    Bds = [(Bd11k*I + Bd12); Bd21k*I + Bd22];
    Cds = [ D11Ik * Cd11 D11Ik * Cd12 ; Dd21k*D11Ik*Cd11 + Cd21 Dd21k*D11Ik*Cd12 + Cd22];
    Dds = [ D11Ik*Dd12; (Dd22+Dd21k*D11Ik*Dd12)];
end

swVecOld = swVec;


    x           = Ads*x_old  + Bds*u(nsw+1:end);  x_old(1:nrSt) = x(1:nrSt);                                                   
    y(1:nrOut)  = Cds*x      + Dds*u(nsw+1:end);        


    is = y(1:nsw)./kb'; %Calculate switch currents


    for i = ncb:nsw

        if(i > ncb) %Breakers

            if(swVec(i)==1 && (is(i) < 0 || y(i) < 0 ))
                swVec(i) = 0; %Open
            end

            if(swVec(i)==0 && y(i) > 0)
                swVec(i) = 1; %Close
            end
        end

    end


    status(1:nsw) = swVec(1:nsw);

end

== matlab function HVDCMMCInterconnection/DQn->ABC ==
  settings: updateMethod=DISCRETE
  data: Xdcpnz_c input; tho input; Xabc output; N parameter
%function abc = Mult(Z0,Zdp,Zqp,Zdn,Zqn,Zdz,Zqz,th, N)
function Xabc = dqn2abc(Xdcpnz_c,tho,N)

    persistent Sas;
    persistent Ssa;

    if(isempty(Sas)) 
        a = -0.5+0.866i;
        a2 = -0.5-0.866i;
        Sas = [1,a,a2;1,a2,a;1,1,1]/3;
        Ssa = eye(3)/(Sas);
    end

    Xabc = zeros(3,1);

    for i = 1 : N+1
    
    
        if(i>1)
            h = i-1;
    
            th = h*tho;
        
            mag_p = abs(Xdcpnz_c(1,i));
            ang_p = angle(Xdcpnz_c(1,i));
            mag_n = abs(Xdcpnz_c(2,i));
            ang_n = angle(Xdcpnz_c(2,i));
            mag_z = abs(Xdcpnz_c(3,i));
            ang_z = angle(Xdcpnz_c(3,i));
            
            abc3p = mag_p*[sin(th+ang_p) ; sin(th+ang_p-2*pi/3) ; sin(th+ang_p+2*pi/3) ];
            abc3n = mag_n*[sin(th+ang_n) ; sin(th+ang_n+2*pi/3) ; sin(th+ang_n-2*pi/3) ];
            abc3z = mag_z*[sin(th+ang_z) ; sin(th+ang_z)        ; sin(th+ang_z)  ];
        
            Xabc = Xabc + abc3p+abc3n+abc3z;
        else
            Xabc = Xabc + real(Ssa*(Xdcpnz_c(:,1)));
        
        end
    
        
    end

end

== matlab function HVDCMMCInterconnection/MATLAB Function1 ==
  data: u input; y output size=33 [1..100]; Ad parameter; Bd parameter; Cd parameter; Dd parameter; dt parameter; nsw parameter; InitVec parameter; bvec input
function y = DSS(u, Ad, Bd, Cd, Dd, dt, nsw, InitVec, bvec)

% INIT
x = zeros(size(Ad,1),1);
y = zeros(size(Cd,1),1);
%bvec_old = zeros(2,1);

persistent Ad11;
persistent Ad12;
persistent Ad21;
persistent Ad22;

persistent Bd11;
persistent Bd12;
persistent Bd21;
persistent Bd22;
persistent Cd11;
persistent Cd12;
persistent Cd21;
persistent Cd22;
persistent Dd11;
persistent Dd12;
persistent Dd21;
persistent Dd22;

persistent Ads;
persistent Bds;
persistent Cds;
persistent Dds;

persistent x_old;
persistent bvec_old;

persistent nrSt;
persistent nrOut;

    
    if(isempty(x_old))

        nrSt = size(Ad,1);
        nrOut = size(Cd,1);

        % swFlag = 0;
        % 
        % arows = size(Ad,1)/3; %signal size
        % acols = size(Ad,2)/3; %signal size
        % 
        % brows = size(Bd,1)/3; %signal size
        % bcols = size(Bd,2)/3; %signal size
        % 
        % crows = size(Cd,1)/3; %signal size
        % ccols = size(Cd,2)/3; %signal size
        % 
        % drows = size(Dd,1)/3; %signal size
        % dcols = size(Dd,2)/3; %signal size
        
        Ad11 = Ad(1:nsw,1:nsw);        if(isempty(Ad11)) Ad11 = zeros(3,3); end
        Ad12 = Ad(1:nsw,nsw+1:end);    if(isempty(Ad12)) Ad12 = zeros(3,3); end
        Ad21 = Ad(nsw+1:end,1:nsw);    if(isempty(Ad21)) Ad21 = zeros(3,3); end
        Ad22 = Ad(nsw+1:end,nsw+1:end); if(isempty(Ad22)) Ad22 = zeros(3,3); end
        
        Bd11 = Bd(1:nsw,1:nsw);        if(isempty(Bd11)) Bd11 = zeros(3,3); end
        Bd12 = Bd(1:nsw,nsw+1:end);    if(isempty(Bd12)) Bd12 = zeros(3,3); end
        Bd21 = Bd(nsw+1:end,1:nsw);    if(isempty(Bd21)) Bd21 = zeros(3,3); end
        Bd22 = Bd(nsw+1:end,nsw+1:end); if(isempty(Bd22)) Bd22 = zeros(3,size(Bd,2)-nsw); end
        
        Cd11 = Cd(1:nsw,1:nsw);        if(isempty(Cd11)) Cd11 = zeros(3,3); end
        Cd12 = Cd(1:nsw,nsw+1:end);    if(isempty(Cd12)) Cd12 = zeros(3,3); end
        Cd21 = Cd(nsw+1:end,1:nsw);    if(isempty(Cd21)) Cd21 = zeros(3,3); end
        Cd22 = Cd(nsw+1:end,nsw+1:end); if(isempty(Cd22)) Cd22 = zeros(size(Cd,1)-nsw,size(Cd,2)); end
        
        Dd11 = Dd(1:nsw,1:nsw);        if(isempty(Dd11)) Dd11 = zeros(3,3); end
        Dd12 = Dd(1:nsw,nsw+1:end);    if(isempty(Dd12)) Dd12 = zeros(3,3); end
        Dd21 = Dd(nsw+1:end,1:nsw);    if(isempty(Dd21)) Dd21 = zeros(3,3); end
        Dd22 = Dd(nsw+1:end,nsw+1:end); if(isempty(Dd22)) Dd22 = zeros(3,3); end
        
        x_old = zeros(size(Ad,1),1);
        bvec_old = bvec;     

        kb1 = 1e6*abs(1-bvec(1))+0.01*abs(0-bvec(1));
        kb2 = 1e6*abs(1-bvec(2))+0.01*abs(0-bvec(2));

        Dd11k = [Dd11(:,1:3)/kb1 Dd11(:,4:6)/kb2];
        D11Ik = eye(nsw)/(eye(nsw) - Dd11k);
        Dd21k = [Dd21(:,1:3)/kb1 Dd21(:,4:6)/kb2];
        
        E = D11Ik * Cd11;
        F = D11Ik * Cd12;
        I = D11Ik*Dd12;
      
        
        Bd11k = [Bd11(:,1:3)/kb1 Bd11(:,4:6)/kb2];
        Bd21k = [Bd21(:,1:3)/kb1 Bd21(:,4:6)/kb2];

        Ads = [Ad11+Bd11k*E Ad12+Bd11k*F ; Ad21+Bd21k*E Ad22+Bd21k*F ];
        Bds = [(Bd11k*I + Bd12); Bd21k*I + Bd22];
        Cds = [ D11Ik * Cd11 D11Ik * Cd12 ; Dd21k*D11Ik*Cd11 + Cd21 Dd21k*D11Ik*Cd12 + Cd22];
        Dds = [ D11Ik*Dd12; (Dd22+Dd21k*D11Ik*Dd12)];
    
    end


    if(any(bvec_old ~= bvec))
        kb1 = 1e6*abs(1-bvec(1))+0.01*abs(0-bvec(1));
        kb2 = 1e6*abs(1-bvec(2))+0.01*abs(0-bvec(2));

        Dd11k = [Dd11(:,1:3)/kb1 Dd11(:,4:6)/kb2];
        D11Ik = eye(nsw)/(eye(nsw) - Dd11k);
        Dd21k = [Dd21(:,1:3)/kb1 Dd21(:,4:6)/kb2];
        
        E = D11Ik * Cd11;
        F = D11Ik * Cd12;
        I = D11Ik*Dd12;
      
        
        Bd11k = [Bd11(:,1:3)/kb1 Bd11(:,4:6)/kb2];
        Bd21k = [Bd21(:,1:3)/kb1 Bd21(:,4:6)/kb2];

        Ads = [Ad11+Bd11k*E Ad12+Bd11k*F ; Ad21+Bd21k*E Ad22+Bd21k*F ];
        Bds = [(Bd11k*I + Bd12); Bd21k*I + Bd22];
        Cds = [ D11Ik * Cd11 D11Ik * Cd12 ; Dd21k*D11Ik*Cd11 + Cd21 Dd21k*D11Ik*Cd12 + Cd22];
        Dds = [ D11Ik*Dd12; (Dd22+Dd21k*D11Ik*Dd12)];
    end


    x = Ads*x_old   + Bds*u(nsw+1:end);                                                     
    y(1:nrOut) = Cds*x       + Dds*u(nsw+1:end);        



    %OLD
    x_old(1:nrSt) = x(1:nrSt);
    bvec_old(1:2) = bvec(1:2);





end

== matlab function HVDCMMCInterconnection/MATLAB Function ==
  data: usw output; Id input; status output; Vd input
function [usw, status]   = DFcn(Id, Vd)

    persistent SW;
    
    if(isempty(SW)) SW = 1; end
    
    
    if(Id<=0 && SW == 1)
    
        SW = 0;
    elseif( (Id>0 && SW == 0) || (Vd > 0.7 && SW == 0 && Id>eps) )
        SW = 1;
    end
    
    status = SW;
    usw = Vd;

end

== matlab function HVDCMMCInterconnection/MATLAB Function2 ==
  data: Usm input; Uref input; UDt output; Stt output; Ip input; Ic input; UDb output; Stb output; IDt output; IDb output; Vbl output; Ts parameter; D_R parameter; D_Rs parameter; Nb_SM parameter; C parameter; Vin output
function [UDt, Stt, UDb, Stb, IDt, IDb, Vbl, Vin]   = DFcn(Usm, Uref, Ip, Ic, Ts, D_R, D_Rs, Nb_SM, C)

    UDt = 0; UDb = 0; Stt = 0; Stb = 0;

    Ib    = 0;
    Vbl = 0;
    Vin = 0;
    IDt = 0;
    IDb = 0;
    
    persistent timer;
    persistent Usm_old;
    persistent Ip_old;
    persistent Ic_old;
    persistent SWt;
    persistent SWb;

    persistent Uc_old;
    persistent Uc;
    persistent x_old;
    persistent Req;
    
    if(isempty(timer)) 
        timer = 0; 
        Usm_old = 0;
        Ip_old = 0;
        Ic_old = 0;
        SWt = 0;
        SWb = 0;
        Uc_old = 0;
        Uc = 0;
        x_old = 0;
        Req = D_R*D_Rs/(D_R+D_Rs);
    end
    
    timer = timer + Ts;

%%%%%%%%%%%%%%% Calc Vin & Vbl %%%%%%%%%%%%%%%
    %x = Nb_SM*(Ip_old*Uref(1)+Ic_old*Uref(2))/(C*Nb_SM);
    x = Nb_SM*(Ip*Uref(1)+Ic*Uref(2))/(C*Nb_SM);

    Uc = (Ts/2)*(x+x_old) + Uc_old;
    
    Vin = Uc*Uref(1)*Nb_SM;
    Vbl = Uc*Uref(2)*Nb_SM;


    x_old = x;
    Uc_old = Uc;
%%%%%%%%%%%%%%%%%%%%%%%%%%%%%%


    Ib = Ip-D_Rs/(D_R+D_Rs)*Ic;


    if(Uref(2) > 0)

        if(Ic < 0)
            UDt = Usm - Vbl;
        else
            UDt = Ic*Req;
        end
    
        if(Ib > 0)
            UDb = -Usm;
        else
            UDb = -Ib*Req;
        end

        1==1;
    
        if(-0.0001 + D_Rs/(D_R+D_Rs)*Ic_old <= 0 && SWt == 1)
            SWt = 0;
        elseif(-0.0001 + D_Rs/(D_R+D_Rs)*Ic > 0 && SWt == 0) 
            SWt = 1;
        end
    
        if(Ib<=0 && SWb == 0 && SWt == 0)
            SWb = 1;
        elseif( (Ib > -eps && SWb == 1 && Vbl > 0 && Ip < 0))
            SWb = 0;
        end

    else
        UDt =  Ip*(D_Rs/2)*D_R/(D_Rs/2+D_R);
        UDb = -UDt;


        if((0.1+Ib<=0 || Ip<0) && SWb == 0)
            SWb = 1;
            SWt = 0;
        elseif( (Ip>0 || -0.1 + Ic >= 0) && SWb == 1)
            SWb = 0;
            SWt = 1;
        end


    end




    IDt = SWt * UDt / D_R;
    if(IDt<0) IDt = 0; end

    IDb = SWb * UDb / D_R;
    if(IDb<0) IDb = 0; end


    Usm_old = Usm;
    Ip_old = Ip;
    Ic_old = Ic;



    Stt =  SWt;
    Stb = SWb;

end


    % if(SWt>0.5)
    %     IDt = UDt / D_R;
    %     if(IDt<0) IDt = 0; end
    % else
    %     IDt = 0;
    % end
    % 
    % if(SWb>0.5)
    %     IDb = UDb / D_R;
    %     if(IDb<0) IDb = 0; end
    % else
    %     IDb = 0;
    % end


    % persistent SW;
    % 
    % if(isempty(SW)) SW = 1; end
    % 
    % 
    % if(Id<=0 && SW == 1)
    % 
    %     SW = 0;
    % elseif( (Id>0 && SW == 0) || (Vd > 0 && SW == 0 && Id>eps) )
    %     SW = 1;
    % end
    % 
    % status = SW;
    % usw = Vd;

== matlab function HVDCMMCInterconnection/MATLAB Function3 ==
  data: u input; y output [1..100]; Ad parameter; Bd parameter; Cd parameter; Dd parameter; swOnRes parameter; swOffRes parameter; swType parameter; brkVec input
function y  = fDSS(u, Ad, Bd, Cd, Dd, swOnRes, swOffRes, swType, brkVec)

% INIT
x = zeros(size(Ad,1),1);
y = zeros(size(Cd,1),1);

persistent Ad11;
persistent Ad12;
persistent Ad21;
persistent Ad22;

persistent Bd11;
persistent Bd12;
persistent Bd21;
persistent Bd22;
persistent Cd11;
persistent Cd12;
persistent Cd21;
persistent Cd22;
persistent Dd11;
persistent Dd12;
persistent Dd21;
persistent Dd22;

persistent Ads;
persistent Bds;
persistent Cds;
persistent Dds;

persistent x_old;
persistent swVec;
persistent swVecOld;

persistent nrSt;
persistent nrOut;

persistent nsw;
persistent ncb;
persistent npe;

persistent kb;


if(isempty(x_old))
    nrSt = size(Ad,1);
    nrOut = size(Cd,1);

    ncb = sum(swType==1) + sum(swType==2);
    npe = sum(swType==3);
    nsw = ncb + npe;
    
    Ad11 = Ad(1:nsw,1:nsw);         if(isempty(Ad11)) Ad11 = zeros(3,3); end
    Ad12 = Ad(1:nsw,nsw+1:end);     if(isempty(Ad12)) Ad12 = zeros(3,3); end
    Ad21 = Ad(nsw+1:end,1:nsw);     if(isempty(Ad21)) Ad21 = zeros(3,3); end
    Ad22 = Ad(nsw+1:end,nsw+1:end); if(isempty(Ad22)) Ad22 = zeros(3,3); end

    Bd11 = Bd(1:nsw,1:nsw);         if(isempty(Bd11)) Bd11 = zeros(3,3); end
    Bd12 = Bd(1:nsw,nsw+1:end);     if(isempty(Bd12)) Bd12 = zeros(3,3); end
    Bd21 = Bd(nsw+1:end,1:nsw);     if(isempty(Bd21)) Bd21 = zeros(3,3); end
    Bd22 = Bd(nsw+1:end,nsw+1:end); if(isempty(Bd22)) Bd22 = zeros(3,size(Bd,2)-nsw); end

    Cd11 = Cd(1:nsw,1:nsw);         if(isempty(Cd11)) Cd11 = zeros(3,3); end
    Cd12 = Cd(1:nsw,nsw+1:end);     if(isempty(Cd12)) Cd12 = zeros(3,3); end
    Cd21 = Cd(nsw+1:end,1:nsw);     if(isempty(Cd21)) Cd21 = zeros(3,3); end
    Cd22 = Cd(nsw+1:end,nsw+1:end); if(isempty(Cd22)) Cd22 = zeros(size(Cd,1)-nsw,size(Cd,2)); end

    Dd11 = Dd(1:nsw,1:nsw);         if(isempty(Dd11)) Dd11 = zeros(3,3); end
    Dd12 = Dd(1:nsw,nsw+1:end);     if(isempty(Dd12)) Dd12 = zeros(3,3); end
    Dd21 = Dd(nsw+1:end,1:nsw);     if(isempty(Dd21)) Dd21 = zeros(3,3); end
    Dd22 = Dd(nsw+1:end,nsw+1:end); if(isempty(Dd22)) Dd22 = zeros(3,3); end

    x_old = zeros(size(Ad,1),1);

    swVec = [brkVec; zeros(nsw - ncb,1) ]; 
    swVecOld = zeros(nsw,1); 

    kb = swOffRes.*abs(1-swVec)+swOnRes.*abs(0-swVec);

    Dd11k = zeros(size(Dd11)); for i = 1 : nsw, Dd11k(:,i) = Dd11(:,i)/kb(i); end
    D11Ik = eye(nsw)/(eye(nsw) - Dd11k);

    Dd21k = zeros(size(Dd21)); for i = 1 : nsw, Dd21k(:,i) = Dd21(:,i)/kb(i);  end

    E = D11Ik * Cd11;
    F = D11Ik * Cd12;
    I = D11Ik*Dd12;

    Bd11k = zeros(size(Bd11)); for i = 1 : nsw, Bd11k(:,i) = Bd11(:,i)/kb(i);  end
    Bd21k = zeros(size(Bd21)); for i = 1 : nsw, Bd21k(:,i) = Bd21(:,i)/kb(i);  end

    Ads = [Ad11+Bd11k*E Ad12+Bd11k*F ; Ad21+Bd21k*E Ad22+Bd21k*F ];
    Bds = [(Bd11k*I + Bd12); Bd21k*I + Bd22];
    Cds = [ D11Ik * Cd11 D11Ik * Cd12 ; Dd21k*D11Ik*Cd11 + Cd21 Dd21k*D11Ik*Cd12 + Cd22];
    Dds = [ D11Ik*Dd12; (Dd22+Dd21k*D11Ik*Dd12)];

end

%is = zeros(nsw,1);

swVec(1:ncb) = brkVec(1:ncb);

if(any(swVecOld ~= swVec))

    kb = swOffRes.*abs(1-swVec)+swOnRes.*abs(0-swVec);
    Dd11k = zeros(size(Dd11)); for i = 1 : nsw, Dd11k(:,i) = Dd11(:,i)/kb(i); end
    D11Ik = eye(nsw)/(eye(nsw) - Dd11k);

    Dd21k = zeros(size(Dd21)); for i = 1 : nsw, Dd21k(:,i) = Dd21(:,i)/kb(i);  end

    E = D11Ik * Cd11;
    F = D11Ik * Cd12;
    I = D11Ik * Dd12;

    Bd11k = zeros(size(Bd11)); for i = 1 : nsw, Bd11k(:,i) = Bd11(:,i)/kb(i);  end
    Bd21k = zeros(size(Bd21)); for i = 1 : nsw, Bd21k(:,i) = Bd21(:,i)/kb(i);  end

    Ads = [Ad11+Bd11k*E Ad12+Bd11k*F ; Ad21+Bd21k*E Ad22+Bd21k*F ];
    Bds = [(Bd11k*I + Bd12); Bd21k*I + Bd22];
    Cds = [ D11Ik * Cd11 D11Ik * Cd12 ; Dd21k*D11Ik*Cd11 + Cd21 Dd21k*D11Ik*Cd12 + Cd22];
    Dds = [ D11Ik*Dd12; (Dd22+Dd21k*D11Ik*Dd12)];
end

swVecOld = swVec;


    x           = Ads*x_old  + Bds*u(nsw+1:end);  x_old(1:nrSt) = x(1:nrSt);                                                   
    y(1:nrOut)  = Cds*x      + Dds*u(nsw+1:end);        


    is = y(1:nsw)./kb'; %Calculate switch currents


    for i = ncb:nsw

        if(i > ncb) %Breakers

            if(swVec(i)==1 && (is(i) <= eps))
                swVec(i) = 0; %Open
            end

            if(swVec(i)==0 && y(i) > 0)
                swVec(i) = 1; %Close
            end
        end

    end




end
